simulink model "Test"  (Simulink 7.4)
settings: Solver=ode45  StartTime=0.0  StopTime=10.0  RelTol=1e-3
settings Model: Creator=dread  LastModifiedBy=dread

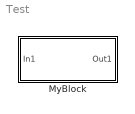
== system Test ==
  MyBlock : Subsystem

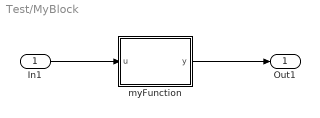
== system Test/MyBlock ==
  In1 : Inport  OutDataType=fixdt(1, 16)  OutScaling=2^0
  myFunction : Stateflow chart
  Out1 : Outport  OutDataType=fixdt(1, 16)  OutScaling=2^0
  wires:
  myFunction/1(y) -> Out1/1
  In1/1 -> myFunction/1(u)

== matlab function MyBlock/myFunction ==
  data: u input double; y output double
function y = fcn(u)
%#eml
%My comment

y = u;
